simulink model "SIM_3DoF_Controller_Test"  (R2024b)
settings: Solver=VariableStepAuto  StartTime=0.0  StopTime=200  RelTol=1e-6
values from neighbouring files (symbols this model uses):
  CL_zero = 0    [my_parameter_search.m]
  delta_maneuver = 1    [my_parameter_search.m]    (also in run_3DoF_SIM_SR22.m = 10; run_3DoF_SIM_SR22_Controller_Test.m = 0)
  deltaE = op_point.Inputs(1).u    [my_parameter_search.m]    (also in run_3DoF_SIM.m = -10; run_3DoF_SIM_SR22.m; run_3DoF_SIM_SR22_Controller_Test.m)
  gravity = 9.807    [run_3DoF_SIM.m]
  J = 30    [run_3DoF_SIM.m]
  M = M - 200    [my_parameter_search.m]
  p_maneuver = 1.5    [my_parameter_search.m]    (also in run_3DoF_SIM_SR22.m; run_3DoF_SIM_SR22_Controller_Test.m)
  rate_maneuver = 7    [my_parameter_search.m]    (also in run_3DoF_SIM_SR22.m; run_3DoF_SIM_SR22_Controller_Test.m)
  states_init = [0 op_point.States.x(2) op_point.States.x(3) op_point.States.x(4) 0 0]    [my_parameter_search.m]    (also in run_3DoF_SIM.m = [0 5000 0 80 0 0]; run_3DoF_SIM_SR22.m; run_3DoF_SIM_SR22_Controller_Test.m)
  t_maneuver = 0    [my_parameter_search.m]    (also in run_3DoF_SIM_SR22.m = 100; run_3DoF_SIM_SR22_Controller_Test.m)
  throttle = op_point.Inputs(2).u    [my_parameter_search.m]    (also in run_3DoF_SIM.m = 0.65; run_3DoF_SIM_SR22.m; run_3DoF_SIM_SR22_Controller_Test.m)
undefined symbols (not defined in the file or in its folder): CD_alpha, CL_alpha, CL_elev, CLEH_alpha, Cm_zero, Cw, down_wash, Sh, Sw, xa, xt
libraries: simulink_extras x7, aerolibatmos2 x2, slpidlib x2
(part 2 of 2)

== system SIM_3DoF_Controller_Test/EofM/Subsystem/Subsystem ==
  x3 : Inport
  gamma : Inport  Port=2
  eta : Inport  Port=3
  Lw : Inport  Port=4
  LT : Inport  Port=5
  D : Inport  Port=6
  Thrust : Inport  Port=7
  1/m : Inport  Port=8
  Add : Sum  Inputs=+-
  Add1 : Sum
  Add2 : Sum
  Cos : Trigonometry  Operator=cos
  Cos1 : Trigonometry  Operator=cos
  Dot Product{,1..4} (5 alike) : DotProduct  OutDataTypeStr=Inherit: Inherit via internal rule
  Sin : Trigonometry
  Sin1 : Trigonometry
  x4_dot : Outport
  wires:
  Add2/1 -> Dot Product4/1
  Cos/1 -> Dot Product1/1
  Add/1 -> Add1/1
  Sin/1 -> Dot Product/1
  Dot Product2/1 -> Add1/2
  LT/1 -> Dot Product2/2
  Dot Product3/1 -> Add2/1
  Dot Product1/1 -> Add/2
  eta/1 -> Cos/1, Sin/1
  Cos1/1 -> Dot Product3/1
  1/m/1 -> Dot Product4/2
  Sin1/1 -> Dot Product2/1
  Dot Product/1 -> Add/1
  Add1/1 -> Add2/2
  gamma/1 -> Sin1/1
  D/1 -> Dot Product1/2
  x3/1 -> Cos1/1
  Lw/1 -> Dot Product/2
  Thrust/1 -> Dot Product3/2
  Dot Product4/1 -> x4_dot/1

== system SIM_3DoF_Controller_Test/EofM/Subsystem/Subsystem1 ==
  x3 : Inport
  gamma : Inport  Port=2
  eta : Inport  Port=3
  Lw : Inport  Port=4
  LT : Inport  Port=5
  D : Inport  Port=6
  Thrust : Inport  Port=7
  1/m : Inport  Port=8
  W : Inport  Port=9
  Add : Sum  Inputs=--
  Add1 : Sum
  Add2 : Sum
  Add3 : Sum
  Cos : Trigonometry
  Cos1 : Trigonometry
  Dot Product{,1..4} (5 alike) : DotProduct  OutDataTypeStr=Inherit: Inherit via internal rule
  Sin : Trigonometry  Operator=cos
  Sin1 : Trigonometry  Operator=cos
  x5_dot : Outport
  wires:
  Dot Product2/1 -> Add1/2
  Add1/1 -> Add2/2
  Sin1/1 -> Dot Product2/1
  Cos1/1 -> Dot Product3/1
  Dot Product/1 -> Add/1
  Add2/1 -> Add3/2
  Cos/1 -> Dot Product1/1
  Sin/1 -> Dot Product/1
  Add/1 -> Add1/1
  Dot Product3/1 -> Add2/1
  1/m/1 -> Dot Product4/2
  Dot Product4/1 -> x5_dot/1
  LT/1 -> Dot Product2/2
  D/1 -> Dot Product1/2
  Dot Product1/1 -> Add/2
  eta/1 -> Cos/1, Sin/1
  gamma/1 -> Sin1/1
  Thrust/1 -> Dot Product3/2
  x3/1 -> Cos1/1
  W/1 -> Add3/1
  Add3/1 -> Dot Product4/1
  Lw/1 -> Dot Product/2

== system SIM_3DoF_Controller_Test/EofM/Subsystem/Subsystem2 ==
  alpha : Inport
  alphaT : Inport  Port=2
  Maero : Inport  Port=3
  Lw : Inport  Port=4
  LT : Inport  Port=5
  xA : Inport  Port=6
  xT : Inport  Port=7
  1/J : Inport  Port=8
  Add : Sum
  Add1 : Sum  Inputs=+-
  Cos : Trigonometry  Operator=cos
  Cos1 : Trigonometry  Operator=cos
  Dot Product{,1..4} (5 alike) : DotProduct  OutDataTypeStr=Inherit: Inherit via internal rule
  x6_dot : Outport
  wires:
  Maero/1 -> Add/1
  Lw/1 -> Dot Product/1
  xA/1 -> Dot Product/2
  alpha/1 -> Cos/1
  Dot Product/1 -> Dot Product1/1
  Cos/1 -> Dot Product1/2
  Dot Product1/1 -> Add/2
  xT/1 -> Dot Product2/2
  Cos1/1 -> Dot Product3/2
  LT/1 -> Dot Product2/1
  Dot Product2/1 -> Dot Product3/1
  alphaT/1 -> Cos1/1
  Add/1 -> Add1/1
  Dot Product3/1 -> Add1/2
  1/J/1 -> Dot Product4/1
  Add1/1 -> Dot Product4/2
  Dot Product4/1 -> x6_dot/1

== system SIM_3DoF_Controller_Test/EofM1/Subsystem/Subsystem ==
  x3 : Inport
  gamma : Inport  Port=2
  eta : Inport  Port=3
  Lw : Inport  Port=4
  LT : Inport  Port=5
  D : Inport  Port=6
  Thrust : Inport  Port=7
  1/m : Inport  Port=8
  Add : Sum  Inputs=+-
  Add1 : Sum
  Add2 : Sum
  Cos : Trigonometry  Operator=cos
  Cos1 : Trigonometry  Operator=cos
  Dot Product{,1..4} (5 alike) : DotProduct  OutDataTypeStr=Inherit: Inherit via internal rule
  Sin : Trigonometry
  Sin1 : Trigonometry
  x4_dot : Outport
  wires:
  Add2/1 -> Dot Product4/1
  Cos/1 -> Dot Product1/1
  Add/1 -> Add1/1
  Sin/1 -> Dot Product/1
  Dot Product2/1 -> Add1/2
  LT/1 -> Dot Product2/2
  Dot Product3/1 -> Add2/1
  Dot Product1/1 -> Add/2
  eta/1 -> Cos/1, Sin/1
  Cos1/1 -> Dot Product3/1
  1/m/1 -> Dot Product4/2
  Sin1/1 -> Dot Product2/1
  Dot Product/1 -> Add/1
  Add1/1 -> Add2/2
  gamma/1 -> Sin1/1
  D/1 -> Dot Product1/2
  x3/1 -> Cos1/1
  Lw/1 -> Dot Product/2
  Thrust/1 -> Dot Product3/2
  Dot Product4/1 -> x4_dot/1

== system SIM_3DoF_Controller_Test/EofM1/Subsystem/Subsystem1 ==
  x3 : Inport
  gamma : Inport  Port=2
  eta : Inport  Port=3
  Lw : Inport  Port=4
  LT : Inport  Port=5
  D : Inport  Port=6
  Thrust : Inport  Port=7
  1/m : Inport  Port=8
  W : Inport  Port=9
  Add : Sum  Inputs=--
  Add1 : Sum
  Add2 : Sum
  Add3 : Sum
  Cos : Trigonometry
  Cos1 : Trigonometry
  Dot Product{,1..4} (5 alike) : DotProduct  OutDataTypeStr=Inherit: Inherit via internal rule
  Sin : Trigonometry  Operator=cos
  Sin1 : Trigonometry  Operator=cos
  x5_dot : Outport
  wires:
  Dot Product2/1 -> Add1/2
  Add1/1 -> Add2/2
  Sin1/1 -> Dot Product2/1
  Cos1/1 -> Dot Product3/1
  Dot Product/1 -> Add/1
  Add2/1 -> Add3/2
  Cos/1 -> Dot Product1/1
  Sin/1 -> Dot Product/1
  Add/1 -> Add1/1
  Dot Product3/1 -> Add2/1
  1/m/1 -> Dot Product4/2
  Dot Product4/1 -> x5_dot/1
  LT/1 -> Dot Product2/2
  D/1 -> Dot Product1/2
  Dot Product1/1 -> Add/2
  eta/1 -> Cos/1, Sin/1
  gamma/1 -> Sin1/1
  Thrust/1 -> Dot Product3/2
  x3/1 -> Cos1/1
  W/1 -> Add3/1
  Add3/1 -> Dot Product4/1
  Lw/1 -> Dot Product/2

== system SIM_3DoF_Controller_Test/EofM1/Subsystem/Subsystem2 ==
  alpha : Inport
  alphaT : Inport  Port=2
  Maero : Inport  Port=3
  Lw : Inport  Port=4
  LT : Inport  Port=5
  xA : Inport  Port=6
  xT : Inport  Port=7
  1/J : Inport  Port=8
  Add : Sum
  Add1 : Sum  Inputs=+-
  Cos : Trigonometry  Operator=cos
  Cos1 : Trigonometry  Operator=cos
  Dot Product{,1..4} (5 alike) : DotProduct  OutDataTypeStr=Inherit: Inherit via internal rule
  x6_dot : Outport
  wires:
  Maero/1 -> Add/1
  Lw/1 -> Dot Product/1
  xA/1 -> Dot Product/2
  alpha/1 -> Cos/1
  Dot Product/1 -> Dot Product1/1
  Cos/1 -> Dot Product1/2
  Dot Product1/1 -> Add/2
  xT/1 -> Dot Product2/2
  Cos1/1 -> Dot Product3/2
  LT/1 -> Dot Product2/1
  Dot Product2/1 -> Dot Product3/1
  alphaT/1 -> Cos1/1
  Add/1 -> Add1/1
  Dot Product3/1 -> Add1/2
  1/J/1 -> Dot Product4/1
  Add1/1 -> Dot Product4/2
  Dot Product4/1 -> x6_dot/1
